simulink model "Modelo_GuPu"  (Simulink 8.3)
settings: Solver=ode45  StartTime=0.0  StopTime=1000  MaxStep=0.1  RelTol=1e-6
settings Model: Creator=Marcelo  LastModifiedBy=lraff  CovSFcnEnable=on
settings DataIOCC: LimitDataPoints=off  SaveOutput=off  SignalLoggingName=sigsOut
settings OptimizationCC: BlockReduction=off  BooleanDataType=off  ExpressionDepthLimit=2147483647
settings DebuggingCC: SaveWithParameterizedLinksMsg=none  SignalResolutionControl=TryResolveAllWithWarning  SolverPrmCheckMsg=none  MultiTaskDSMMsg=warning  MultiTaskCondExecSysMsg=none  FcnCallInpInsideContextMsg=UseLocalSettings  FrameProcessingCompatibilityMsg=error
settings HardwareCC: TargetUnknown=on

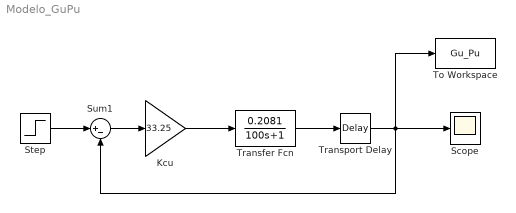
== system Modelo_GuPu ==
  Kcu : Gain  Gain=33.25
  Scope : Scope
      settings: YMin=0.772488  YMax=0.772498
  Step : Step  Time=50  Before=1  SampleTime=0
  Sum1 : Sum  Inputs=|+-  SaturateOnIntegerOverflow=on  InputSameDT=on  OutDataTypeStr=Inherit: Same as first input
  To Workspace : ToWorkspace  VariableName=Gu_Pu  SaveFormat=Structure With Time
  Transfer Fcn : TransferFcn  Numerator=[0.2081]  Denominator=[100 1]
  Transport Delay : TransportDelay  DelayTime=25
  wires:
  Transfer Fcn/1 -> Transport Delay/1
  Transport Delay/1 -> To Workspace/1, Scope/1, Sum1/2
  Kcu/1 -> Transfer Fcn/1
  Sum1/1 -> Kcu/1
  Step/1 -> Sum1/1
